simulink model "unballance_elev"  (R2022b)
settings: Solver=VariableStepAuto  StartTime=0.0  StopTime=10.0  RelTol=1e-3
settings Model: Creator=ohadformanair  LastModifiedBy=ohadformanair

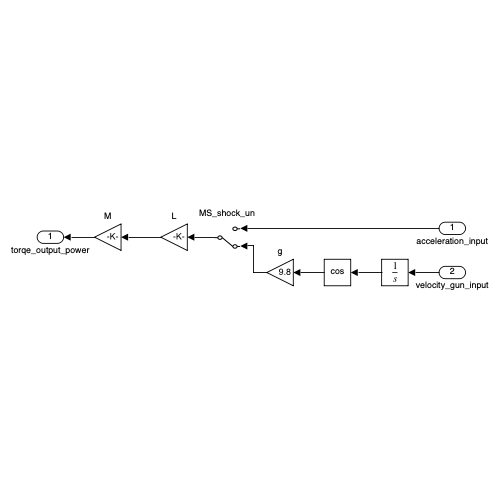
[thumbnail: Simulink's stored preview of the top-level diagram]
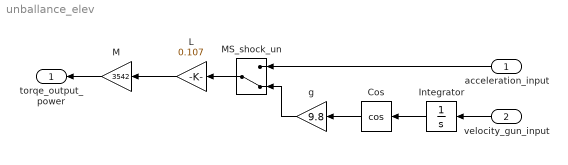
== system unballance_elev ==
  acceleration_input : Inport
  velocity_gun_input : Inport  Port=2
  Cos : Trigonometry  Operator=cos
  Integrator : Integrator
  L : Gain  Gain=0.107
  M : Gain  Gain=3542
  MS_shock_un : ManualSwitch  CurrentSetting=0
  g : Gain  Gain=9.8
  torqe_output_power : Outport
  wires:
  Cos/1 -> g/1
  acceleration_input/1 -> MS_shock_un/1
  MS_shock_un/1 -> L/1
  Integrator/1 -> Cos/1
  L/1 -> M/1
  M/1 -> torqe_output_power/1
  velocity_gun_input/1 -> Integrator/1
  g/1 -> MS_shock_un/2
